simulink model "PID_Controller"  (R2020b)
settings: Solver=VariableStepAuto  StartTime=0.0  StopTime=100  RelTol=1e-3
InitFcn:
  | M = 1000;
  | b = 50;
  | u = 500;
  | Kp=330;
  | Ki=43;
  | Kd=-8;
settings Model: DataDictionary=MBD2_problem3_data.sldd  Creator=Lenovo  LastModifiedBy=Lenovo
settings DataIOCC: SaveOutput=off  SaveTime=off

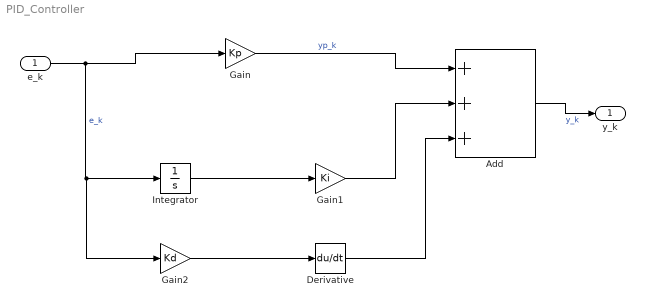
== system PID_Controller ==
  e_k : Inport  OutDataTypeStr=double  PortDimensions=1  SampleTime=0
  Add : Sum  Inputs=+++
  Derivative : Derivative
  Gain : Gain  Gain=Kp
  Gain1 : Gain  Gain=Ki
  Gain2 : Gain  Gain=Kd
  Integrator : Integrator
  y_k : Outport  OutDataTypeStr=double  PortDimensions=1  SampleTime=0
  wires:
  e_k/1 -> Integrator/1, Gain2/1, Gain/1  "e_k"
  Add/1 -> y_k/1  "y_k"
  Gain/1 -> Add/1  "yp_k"
  Gain1/1 -> Add/2
  Integrator/1 -> Gain1/1
  Gain2/1 -> Derivative/1
  Derivative/1 -> Add/3
